simulink model "Es_5"  (R2023b)
settings: Solver=VariableStepAuto  StartTime=0.0  StopTime=15  RelTol=1e-3
libraries: robotmobilelib x1
settings Model: LastModifiedBy=paolo
settings ModelReferenceCC: EnableRefExpFcnMdlSchedulingChecks=on

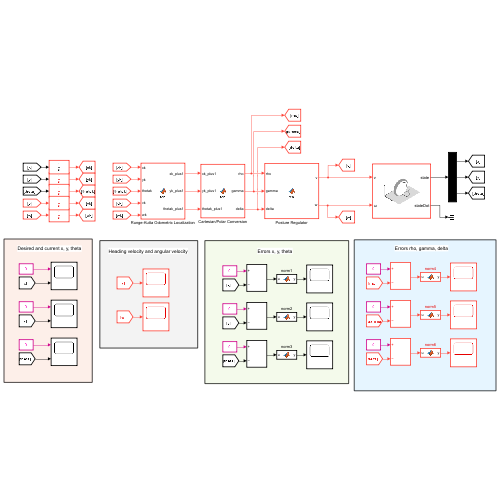
[thumbnail: Simulink's stored preview of the top-level diagram]
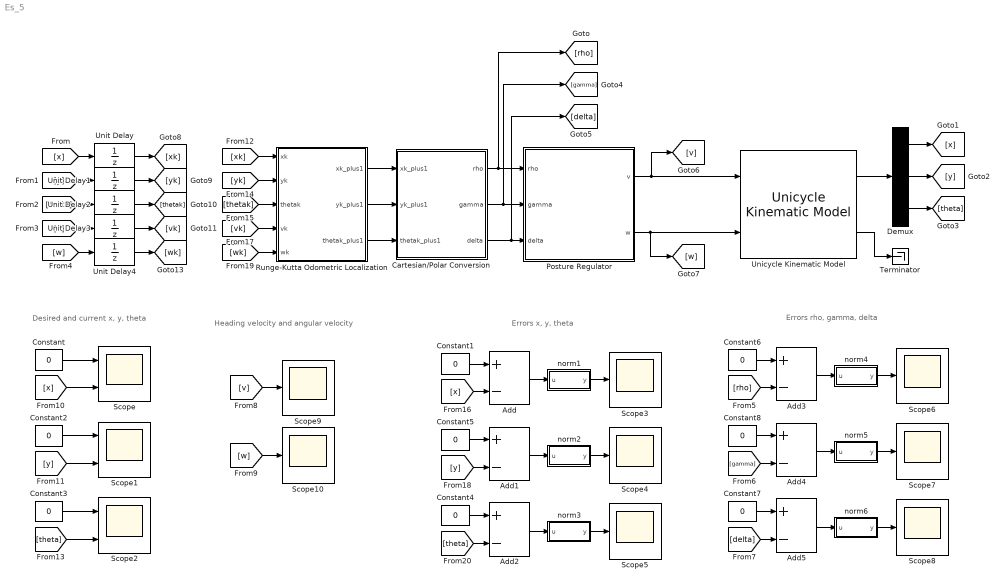
== system Es_5 ==
  note: Errors x, y, theta
  note: Desired and current x, y, theta
  note: Errors rho, gamma, delta
  note: Heading velocity and angular velocity
  Add{,1..5} (6 alike) : Sum  Inputs=+-
  Cartesian/Polar Conversion : MATLAB Function  TreatAsAtomicUnit=on
  Constant{,1..8} (9 alike) : Constant  Value=0
  Demux : Demux  Outputs=3
  Posture Regulator : MATLAB Function  TreatAsAtomicUnit=on
  Runge-Kutta Odometric Localization : MATLAB Function  TreatAsAtomicUnit=on
  Scope : Scope  NumInputPorts=2
  Scope1 : Scope  NumInputPorts=2
  Scope{3..10} (8 alike) : Scope
  Scope2 : Scope  NumInputPorts=2
  Terminator : Terminator
  Unicycle Kinematic Model : robotmobilelib/Unicycle Kinematic Model  VehicleInputs=Vehicle Speed & Heading Angular Velocity  WheelRadius=0.2  WheelSpeedRange=[-Inf Inf]  InitialState=[2; 1; pi/4]  SimulateUsing=Interpreted execution
  Unit Delay{,1..4} (5 alike) : UnitDelay  SampleTime=0.001  HasFrameUpgradeWarning=on
  norm1 : MATLAB Function  TreatAsAtomicUnit=on
  norm2 : MATLAB Function  TreatAsAtomicUnit=on
  norm3 : MATLAB Function  TreatAsAtomicUnit=on
  norm4 : MATLAB Function  TreatAsAtomicUnit=on
  norm5 : MATLAB Function  TreatAsAtomicUnit=on
  norm6 : MATLAB Function  TreatAsAtomicUnit=on
  wires:
  Posture Regulator/1(v) -> [v], Unicycle Kinematic Model/1
  Posture Regulator/2(w) -> Unicycle Kinematic Model/2, [w]
  Demux/3 -> [theta]
  Unicycle Kinematic Model/1 -> Demux/1
  Demux/1 -> [x]
  Demux/2 -> [y]
  [x] -> Add/2
  norm3/1(y) -> Scope5/1
  [theta] -> Add2/2
  Add1/1 -> norm2/1(u)
  Constant4/1 -> Add2/1
  Constant3/1 -> Scope2/1
  norm2/1(y) -> Scope4/1
  [y] -> Add1/2
  Add/1 -> norm1/1(u)
  [x] -> Scope/2
  norm1/1(y) -> Scope3/1
  Add2/1 -> norm3/1(u)
  [theta] -> Scope2/2
  [y] -> Scope1/2
  Constant/1 -> Scope/1
  Constant2/1 -> Scope1/1
  Constant5/1 -> Add1/1
  Constant1/1 -> Add/1
  Cartesian/Polar Conversion/1(rho) -> [rho], Posture Regulator/1(rho)
  Cartesian/Polar Conversion/3(delta) -> [delta], Posture Regulator/3(delta)
  Runge-Kutta Odometric Localization/3(thetak_plus1) -> Cartesian/Polar Conversion/3(thetak_plus1)
  [xk] -> Runge-Kutta Odometric Localization/1(xk)
  [yk] -> Runge-Kutta Odometric Localization/2(yk)
  [thetak] -> Runge-Kutta Odometric Localization/3(thetak)
  [vk] -> Runge-Kutta Odometric Localization/4(vk)
  [wk] -> Runge-Kutta Odometric Localization/5(wk)
  Runge-Kutta Odometric Localization/1(xk_plus1) -> Cartesian/Polar Conversion/1(xk_plus1)
  Runge-Kutta Odometric Localization/2(yk_plus1) -> Cartesian/Polar Conversion/2(yk_plus1)
  Cartesian/Polar Conversion/2(gamma) -> [gamma], Posture Regulator/2(gamma)
  [v] -> Scope9/1
  [w] -> Scope10/1
  Constant8/1 -> Add4/1
  Add4/1 -> norm5/1(u)
  [gamma] -> Add4/2
  Add3/1 -> norm4/1(u)
  [delta] -> Add5/2
  norm5/1(y) -> Scope7/1
  Constant6/1 -> Add3/1
  norm4/1(y) -> Scope6/1
  Constant7/1 -> Add5/1
  [rho] -> Add3/2
  norm6/1(y) -> Scope8/1
  Add5/1 -> norm6/1(u)
  [w] -> Unit Delay4/1
  [y] -> Unit Delay1/1
  [x] -> Unit Delay/1
  [v] -> Unit Delay3/1
  [theta] -> Unit Delay2/1
  Unit Delay/1 -> [xk]
  Unit Delay1/1 -> [yk]
  Unit Delay2/1 -> [thetak]
  Unit Delay3/1 -> [vk]
  Unit Delay4/1 -> [wk]
  Unicycle Kinematic Model/2 -> Terminator/1

== matlab function Es_5/Runge-Kutta Odometric Localization ==
  data: xk_plus1 output; yk_plus1 output; thetak_plus1 output; xk input; yk input; thetak input; vk input; wk input
function [xk_plus1,yk_plus1,thetak_plus1] = fcn(xk,yk,thetak,vk,wk)

Ts=0.001;

xk_plus1=xk+vk*Ts*cos(thetak+(wk*Ts)/2);
yk_plus1=yk+vk*Ts*sin(thetak+(wk*Ts)/2);
thetak_plus1=thetak+wk*Ts;

end

== matlab function Es_5/Posture Regulator ==
  data: rho input; v output; gamma input; delta input; w output
function [v,w] = fcn(rho,gamma,delta)

k1=4;
k2=5;
k3=0.2;

v=k1*rho*cos(gamma);
w=k2*gamma+k1*sin(gamma)*cos(gamma)*(1+(k3*delta)/gamma);

end

== matlab function Es_5/Cartesian//Polar Conversion ==
  data: xk_plus1 input; rho output; yk_plus1 input; thetak_plus1 input; gamma output; delta output
function [rho,gamma,delta] = fcn(xk_plus1,yk_plus1,thetak_plus1)

rho=sqrt(xk_plus1^2+yk_plus1^2);
gamma=atan2(yk_plus1,xk_plus1)-thetak_plus1+pi;
delta=gamma+thetak_plus1;

end

== matlab function Es_5/norm4 ==
  data: u input; y output
function y = norm(u)
y = norm(u);

== matlab function Es_5/norm1 ==
  data: u input; y output
function y = norm(u)
y = norm(u);

== matlab function Es_5/norm2 ==
  data: u input; y output
function y = norm(u)
y = norm(u);

== matlab function Es_5/norm3 ==
  data: u input; y output
function y = norm(u)
y = norm(u);

== matlab function Es_5/norm5 ==
  data: u input; y output
function y = norm(u)
y = norm(u);

== matlab function Es_5/norm6 ==
  data: u input; y output
function y = norm(u)
y = norm(u);
